simulink model "DoubleInvertedPendulum_LQG"  (R2017a)
settings: Solver=VariableStepAuto  StartTime=0.0  StopTime=10.0  RelTol=1e-3
values from neighbouring files (symbols this model uses):
  a = [ 0       1       0       0       0       0 ... (first row only)    [DoubleInvertedPendulum_LQG.m]    (also in TermProject_DoubleInvertedPendulum_LQG_MFile.m)
  b = [ 0       0.8459  0      -2.5204  0      -0.2998 ]'    [DoubleInvertedPendulum_LQG.m]    (also in TermProject_DoubleInvertedPendulum_LQG_MFile.m)
  c = [ 1       0       0       0       0       0 ... (first row only)    [DoubleInvertedPendulum_LQG.m]    (also in TermProject_DoubleInvertedPendulum_LQG_MFile.m)
  d = zeros(3,1)    [DoubleInvertedPendulum_LQG.m]    (also in TermProject_DoubleInvertedPendulum_LQG_MFile.m)
  Kr = lqr(a, b, Q, R)    [DoubleInvertedPendulum_LQG.m]    (also in TermProject_DoubleInvertedPendulum_LQG_MFile.m)
undefined symbols (not defined in the file or in its folder): Ke
settings Model: Creator=abxis  LastModifiedBy=abxis

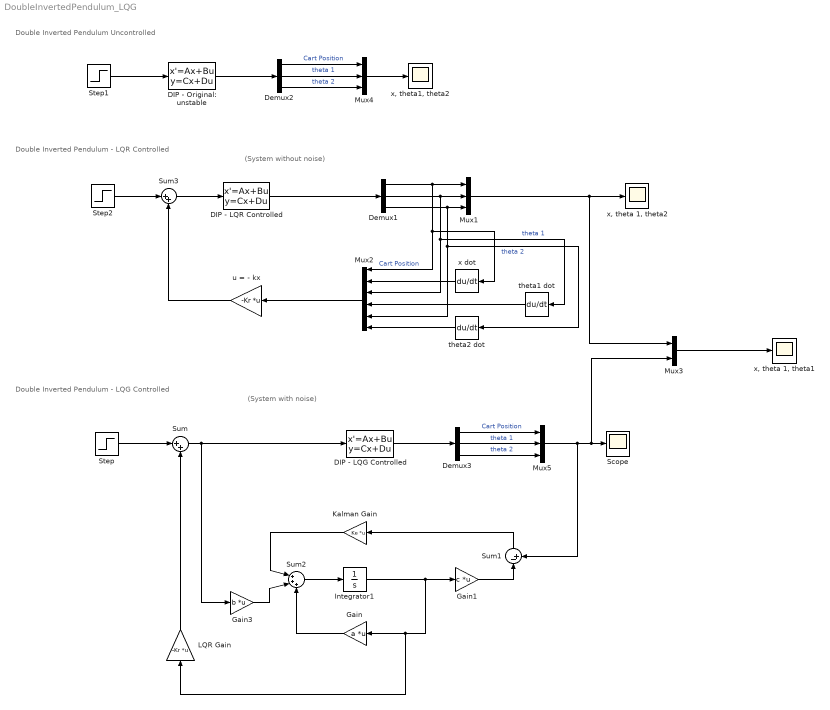
== system DoubleInvertedPendulum_LQG ==
  note: (System with noise)
  note: (System without noise)
  note: Double Inverted Pendulum - LQG Controlled
  note: Double Inverted Pendulum - LQR Controlled
  note: Double Inverted Pendulum Uncontrolled
  " x, theta 1, theta1" : Scope
  " x, theta 1, theta2" : Scope
  DIP - LQG Controlled : StateSpace  A=a  B=b  C=c  D=d  X0=0
  DIP - LQR Controlled : StateSpace  A=a  B=b  C=c  D=d  X0=0
  DIP - Original: unstable : StateSpace  A=a  B=b  C=c  D=d  X0=0
  Demux1 : Demux  Outputs=3
  Demux2 : Demux  Outputs=3
  Demux3 : Demux  Outputs=3
  Gain : Gain  Gain=a  Multiplication=Matrix(K*u)
  Gain1 : Gain  Gain=c  Multiplication=Matrix(K*u)
  Gain3 : Gain  Gain=b  Multiplication=Matrix(K*u)
  Integrator1 : Integrator
  Kalman Gain : Gain  Gain=Ke  Multiplication=Matrix(K*u)
  LQR Gain : Gain  Gain=-Kr  Multiplication=Matrix(K*u)
  Mux1 : Mux  Inputs=3
  Mux2 : Mux  Inputs=6
  Mux3 : Mux  Inputs=2
  Mux4 : Mux  Inputs=3
  Mux5 : Mux  Inputs=3
  Scope : Scope
  Step : Step  Time=0  SampleTime=0
  Step1 : Step  Time=0  SampleTime=0
  Step2 : Step  Time=0  SampleTime=0
  Sum : Sum  Inputs=|++
  Sum1 : Sum  Inputs=|-+
  Sum2 : Sum  Inputs=|+++
  Sum3 : Sum  Inputs=|++
  theta1 dot : Derivative
  theta2 dot : Derivative
  u = - kx : Gain  Gain=-Kr  Multiplication=Matrix(K*u)
  x dot : Derivative
  "x, theta1, theta2" : Scope
  wires:
  Sum/1 -> DIP - LQG Controlled/1, Gain3/1
  Sum2/1 -> Integrator1/1
  Integrator1/1 -> LQR Gain/1, Gain/1, Gain1/1
  Gain1/1 -> Sum1/1
  Sum1/1 -> Kalman Gain/1
  Kalman Gain/1 -> Sum2/1
  Gain/1 -> Sum2/3
  Gain3/1 -> Sum2/2
  LQR Gain/1 -> Sum/2
  Step/1 -> Sum/1
  x dot/1 -> Mux2/2
  Mux2/1 -> u = - kx/1
  Step2/1 -> Sum3/1
  theta2 dot/1 -> Mux2/6
  theta1 dot/1 -> Mux2/4
  Demux1/1 -> Mux2/1, x dot/1, Mux1/1  "Cart Position"
  DIP - LQR Controlled/1 -> Demux1/1
  u = - kx/1 -> Sum3/2
  Demux1/2 -> Mux2/3, theta1 dot/1, Mux1/2  "theta 1"
  Demux1/3 -> Mux2/5, theta2 dot/1, Mux1/3  "theta 2"
  Mux1/1 -> Mux3/1, " x, theta 1, theta2"/1
  Step1/1 -> DIP - Original: unstable/1
  Sum3/1 -> DIP - LQR Controlled/1
  Mux3/1 -> " x, theta 1, theta1"/1
  Demux2/3 -> Mux4/3  "theta 2"
  Demux2/2 -> Mux4/2  "theta 1"
  Demux2/1 -> Mux4/1  "Cart Position"
  DIP - Original: unstable/1 -> Demux2/1
  Mux4/1 -> "x, theta1, theta2"/1
  Demux3/1 -> Mux5/1  "Cart Position"
  DIP - LQG Controlled/1 -> Demux3/1
  Mux5/1 -> Sum1/2, Mux3/2, Scope/1
  Demux3/3 -> Mux5/3  "theta 2"
  Demux3/2 -> Mux5/2  "theta 1"
